simulink model "Three_phase_invertor"  (R2024b)
settings: Solver=VariableStepAuto  StartTime=0.0  StopTime=10.0  RelTol=1e-3
libraries: spsIGBTLib x6, spsThreePhaseVIMeasurementLib x2, spsDCVoltageSourceLib x1, spsGroundLib x1, spsThreePhaseParallelRLCBranchLib x1

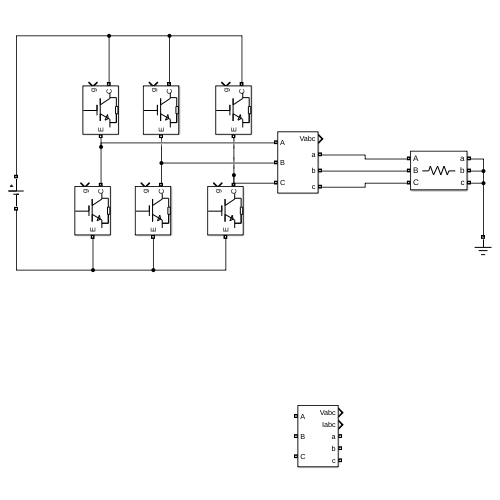
[thumbnail: Simulink's stored preview of the top-level diagram]
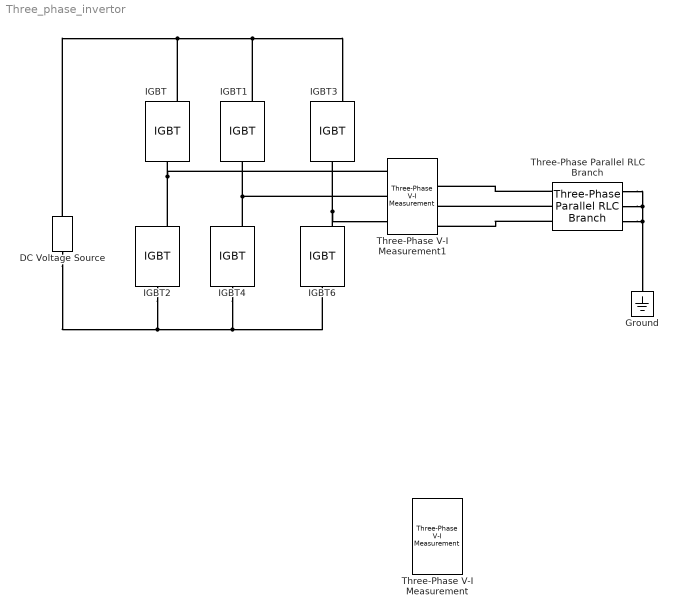
== system Three_phase_invertor ==
  DC Voltage Source : spsDCVoltageSourceLib/DC Voltage Source  Amplitude=100  Measurements=None
  Ground : spsGroundLib/Ground  LConnTagsString=a
  IGBT{,1..4,6} (6 alike) : spsIGBTLib/IGBT  Ron=0.001  Lon=0  Vf=1  Tf=1e-6  Tt=2e-6  IC=0  Rs=1e5  Cs=inf  Measurements=off
  Three-Phase Parallel RLC Branch : spsThreePhaseParallelRLCBranchLib/Three-Phase Parallel RLC Branch  LConnTagsString=A|B|C  RConnTagsString=A|B|C  BranchType=R  Resistance=1  Inductance=1e-3  Capacitance=1e-6  Measurements=None
  Three-Phase V-I Measurement : spsThreePhaseVIMeasurementLib/Three-Phase V-I Measurement  VoltageMeasurement=phase-to-ground  SetLabelV=off  LabelV=Vabc  Vpu=off  VpuLL=off  CurrentMeasurement=yes  SetLabelI=off  LabelI=Iabc  Ipu=off  Pbase=100e6  Vbase=500e3  OutputType=Complex  PhasorSimulation=off  PSBequivalent=0
  Three-Phase V-I Measurement1 : spsThreePhaseVIMeasurementLib/Three-Phase V-I Measurement  VoltageMeasurement=phase-to-ground  SetLabelV=off  LabelV=Vabc  Vpu=off  VpuLL=off  CurrentMeasurement=no  SetLabelI=off  LabelI=Iabc  Ipu=off  Pbase=100e6  Vbase=500e3  OutputType=Complex  PhasorSimulation=off  PSBequivalent=0
  connections:
  DC Voltage Source/RConn1 -- IGBT/LConn1 -- IGBT1/LConn1 -- IGBT3/LConn1
  DC Voltage Source/LConn1 -- IGBT2/RConn1 -- IGBT4/RConn1 -- IGBT6/RConn1
  IGBT2/LConn1 -- Three-Phase V-I Measurement1/LConn1 -- IGBT/RConn1
  IGBT4/LConn1 -- Three-Phase V-I Measurement1/LConn2 -- IGBT1/RConn1
  IGBT6/LConn1 -- Three-Phase V-I Measurement1/LConn3 -- IGBT3/RConn1
  Three-Phase Parallel RLC Branch/LConn1 -- Three-Phase V-I Measurement1/RConn1
  Three-Phase Parallel RLC Branch/LConn2 -- Three-Phase V-I Measurement1/RConn2
  Three-Phase Parallel RLC Branch/LConn3 -- Three-Phase V-I Measurement1/RConn3
  Three-Phase Parallel RLC Branch/RConn1 -- Three-Phase Parallel RLC Branch/RConn2 -- Three-Phase Parallel RLC Branch/RConn3 -- Ground/LConn1
